simulink model "uav_control_ASMC"  (R2023a)
settings: Solver=FixedStepAuto  StartTime=0.0  StopTime=50  FixedStep=1e-3
undefined symbols (not defined in the file): C_SMC, control_form_LagrangeSimplified_forces, D_rot, D_transl, eulerlimit, g, J1, J2, J3, Jr, k1, k2, k3, k_phi, K_SMC, k_theta, m, Matrix_Force2angular_velocity, R
libraries: simulink x18, control_form_LagrangeSimplified x1
settings Model: Creator=Alex  LastModifiedBy=Alex

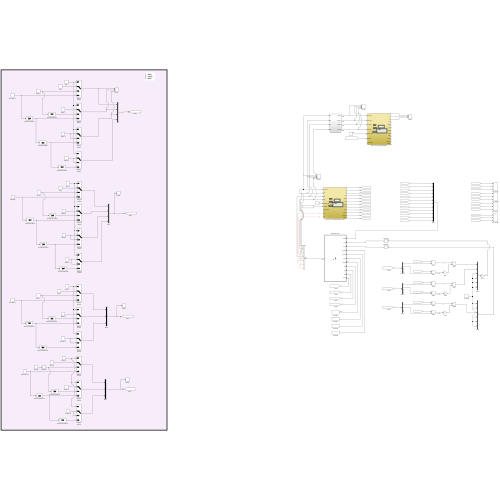
[thumbnail: Simulink's stored preview of the top-level diagram]
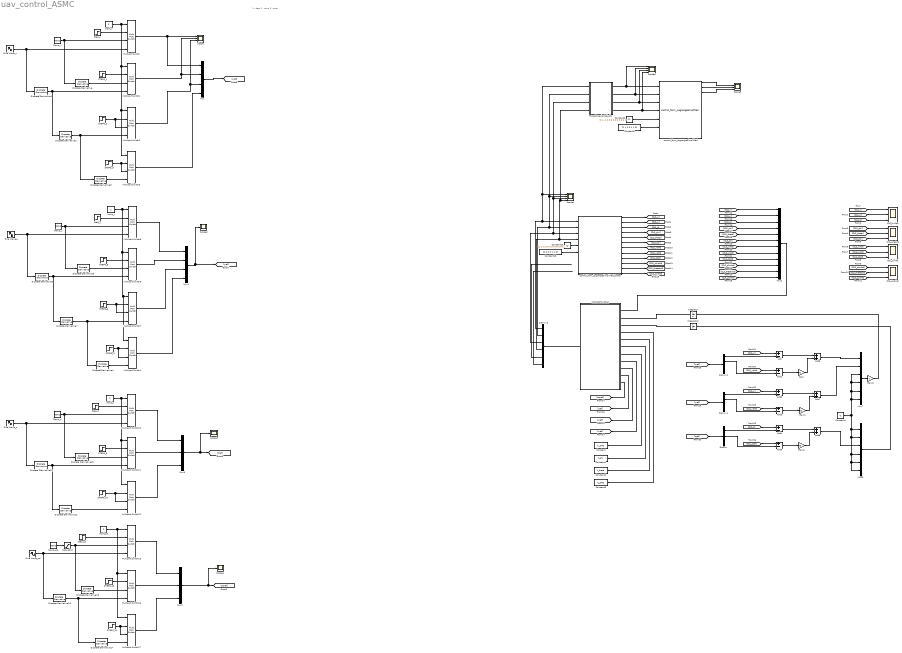
== system uav_control_ASMC ==
  note: 1 - step
      | 2 - ramp
      | 3 - else
  Add{,1..5} (6 alike) : Sum  Inputs=+-
  Add6 : Sum
  Add7 : Sum
  Add8 : Sum
  CNL_AngPos : Scope  NumInputPorts=3
  CNL_AngVel : Scope  NumInputPorts=3
  CNL_LinPos : Scope  NumInputPorts=3
  CNL_LinVel : Scope  NumInputPorts=3
  Constant : Constant  Value=K_SMC
  Constant1 : Constant  Value=k_phi
  Constant18 : Constant  Value=[1 0 0 0 1 1 0]
  Constant19 : Constant  Value=[1 1 -1 0 0 0 0 0 0 0 0 0 ]
  Constant2 : Constant  Value=k_theta
  Constant3 : Constant  Value=C_SMC
  Constant4 : Constant  Value=0
  Constant5 : Constant  Value=[1 1 0 0 1 1 0]
  Constant6 : Constant  Value=[1 1 -1 0 0 0 0 0 0 0 0 0 ]
  Demux : Demux  Outputs=3
  Demux1 : Demux
  Demux2 : Demux
  Demux3 : Demux  Outputs=6
  Discrete Derivative{,1..7,10..12,15..17} (14 alike) : simulink/Discrete/Discrete Derivative  gainval=1.0  ICPrevScaledInput=0.0  OutMin=[]  OutMax=[]  OutDataType=fixdt(1, 16)  OutScaling=2^-10  DoSatur=off
  Force2AngularVelocity : Subsystem
  Gain : Gain  Gain=k1
  Gain1 : Gain  Gain=k2
  Gain2 : Gain  Gain=k3
  Gain3 : Gain  Gain=-1
  Input_psi : Constant
  Input_x : Constant
  Input_y : Constant
  Input_z : Constant
  Integrator : Integrator
  Integrator1 : Integrator
  MATLAB Function : MATLAB Function  TreatAsAtomicUnit=on
  Multiport Switch{,1..7,10..12,15..17} (14 alike) : MultiPortSwitch  SaturateOnIntegerOverflow=off  InputSameDT=off
  Mux : Mux
  Mux1 : Mux
  Mux2 : Mux  Inputs=12
  Mux3 : Mux  Inputs=3
  Mux5 : Mux  Inputs=3
  Mux7 : Mux  Inputs=6
  Mux8 : Mux  Inputs=6
  Ramp_psi : simulink/Sources/Ramp  slope=0.2  start=0  InitialOutput=0
  Ramp_x : simulink/Sources/Ramp  slope=1  start=0  InitialOutput=1
  Ramp_y : simulink/Sources/Ramp  slope=1  start=0  InitialOutput=0
  Ramp_z : simulink/Sources/Ramp  slope=-5  start=0  InitialOutput=0
  STEP0_{1..6,9..10,13..14} (10 alike) : Step  Time=0  After=0  SampleTime=0
  Saturation : Saturate  UpperLimit=pi  LowerLimit=-pi
  Scope : Scope  NumInputPorts=3
  Scope1 : Scope  NumInputPorts=4
  Scope2 : Scope
  Scope3 : Scope
  Scope4 : Scope
  Scope5 : Scope  NumInputPorts=3
  Scope6 : Scope  NumInputPorts=4
  Sine Wave_psi : Sin  SampleTime=0
  Sine Wave_x : Sin  Frequency=0.5  SampleTime=0
  Sine Wave_y : Sin  Amplitude=3  Bias=5  SampleTime=0
  Sine Wave_z : Sin  Amplitude=3  Bias=-5  SampleTime=0
  Step_psi : Step  Time=0  SampleTime=0
  Step_x : Step  Time=0  After=5  SampleTime=0
  Step_y : Step  Time=0  After=5  SampleTime=0
  Step_z : Step  Time=0  After=-7  SampleTime=0
  control_form_LagrangeSimplified : control_form_LagrangeSimplified/control_form_LagrangeSimplified  SystemSampleTime=-1  VariantActivationTime=update diagram  Latency=0  AutoFrameSizeCalculation=off
  control_form_LagrangeSimplified_forces : Subsystem  AncestorBlock=control_form_LagrangeSimplified_forces/control_form_LagrangeSimplified_forces
  wires:
  Step_x/1 -> Multiport Switch/2
  Mux/1 -> [xref]
  Mux1/1 -> [yref], Scope2/1
  Step_psi/1 -> Multiport Switch15/2
  Mux3/1 -> Scope4/1, [psiref]
  Ramp_x/1 -> Discrete Derivative/1, Multiport Switch/3
  Sine Wave_x/1 -> Multiport Switch/4, Discrete Derivative1/1
  Input_x/1 -> Multiport Switch3/1, Multiport Switch2/1, Multiport Switch1/1, Multiport Switch/1
  STEP0_1/1 -> Multiport Switch1/2
  Discrete Derivative/1 -> Multiport Switch1/3
  Discrete Derivative1/1 -> Multiport Switch1/4, Discrete Derivative2/1
  STEP0_2/1 -> Multiport Switch2/3, Multiport Switch2/2
  Discrete Derivative2/1 -> Discrete Derivative3/1, Multiport Switch2/4
  Multiport Switch/1 -> Mux/1, Scope/1
  Multiport Switch1/1 -> Mux/2, Scope/2
  Multiport Switch2/1 -> Mux/3, Scope/3
  Multiport Switch7/1 -> Mux1/3
  Multiport Switch6/1 -> Mux1/2
  Multiport Switch5/1 -> Mux1/1
  Discrete Derivative7/1 -> Discrete Derivative4/1, Multiport Switch7/4
  STEP0_6/1 -> Multiport Switch7/2, Multiport Switch7/3
  Discrete Derivative6/1 -> Discrete Derivative7/1, Multiport Switch6/4
  Discrete Derivative5/1 -> Multiport Switch6/3
  STEP0_5/1 -> Multiport Switch6/2
  Input_y/1 -> Multiport Switch4/1, Multiport Switch7/1, Multiport Switch6/1, Multiport Switch5/1
  Sine Wave_y/1 -> Discrete Derivative6/1, Multiport Switch5/4
  Ramp_y/1 -> Multiport Switch5/3, Discrete Derivative5/1
  Step_y/1 -> Multiport Switch5/2
  Step_z/1 -> Multiport Switch10/2
  Ramp_z/1 -> Discrete Derivative10/1, Multiport Switch10/3
  Sine Wave_z/1 -> Multiport Switch10/4, Discrete Derivative11/1
  Input_z/1 -> Multiport Switch12/1, Multiport Switch11/1, Multiport Switch10/1
  STEP0_9/1 -> Multiport Switch11/2
  Discrete Derivative10/1 -> Multiport Switch11/3
  Discrete Derivative11/1 -> Multiport Switch11/4, Discrete Derivative12/1
  STEP0_10/1 -> Multiport Switch12/3, Multiport Switch12/2
  Discrete Derivative12/1 -> Multiport Switch12/4
  Multiport Switch10/1 -> Mux5/1
  Multiport Switch11/1 -> Mux5/2
  Multiport Switch12/1 -> Mux5/3
  Mux5/1 -> Scope3/1, [zref]
  Input_psi/1 -> Multiport Switch17/1, Multiport Switch16/1, Multiport Switch15/1
  Ramp_psi/1 -> Saturation/1
  Saturation/1 -> Discrete Derivative15/1, Multiport Switch15/3
  Sine Wave_psi/1 -> Discrete Derivative16/1, Multiport Switch15/4
  STEP0_13/1 -> Multiport Switch16/2
  Discrete Derivative15/1 -> Multiport Switch16/3
  Discrete Derivative16/1 -> Discrete Derivative17/1, Multiport Switch16/4
  STEP0_14/1 -> Multiport Switch17/3, Multiport Switch17/2
  Discrete Derivative17/1 -> Multiport Switch17/4
  Multiport Switch15/1 -> Mux3/1
  Multiport Switch16/1 -> Mux3/2
  Multiport Switch17/1 -> Mux3/3
  control_form_LagrangeSimplified_forces/1(x) -> [CLS_x]
  control_form_LagrangeSimplified_forces/2(y) -> [CLS_y]
  control_form_LagrangeSimplified_forces/3(z) -> [CLS_z]
  control_form_LagrangeSimplified_forces/4(phi) -> [CLS_phi]
  control_form_LagrangeSimplified_forces/5(theta) -> [CLS_theta]
  control_form_LagrangeSimplified_forces/6(psi) -> [CLS_psi]
  control_form_LagrangeSimplified_forces/7(xdot) -> [CLS_xdot]
  control_form_LagrangeSimplified_forces/8(ydot) -> [CLS_ydot]
  control_form_LagrangeSimplified_forces/9(zdot) -> [CLS_zdot]
  control_form_LagrangeSimplified_forces/10(phidot) -> [CLS_phidot]
  control_form_LagrangeSimplified_forces/11(thetadot) -> [CLS_thetadot]
  control_form_LagrangeSimplified_forces/12(psidot) -> [CLS_psidot]
  [CLS_x] -> Mux2/1
  [CLS_x] -> CNL_LinPos/1
  [CLS_y] -> Mux2/2
  [CLS_xdot] -> CNL_LinVel/1
  [CLS_psidot] -> Mux2/12
  [CLS_zdot] -> Mux2/9
  [CLS_thetadot] -> CNL_AngVel/2
  [CLS_phi] -> CNL_AngPos/1
  [CLS_ydot] -> CNL_LinVel/2
  [CLS_psidot] -> CNL_AngVel/3
  Mux2/1 -> MATLAB Function/1(states)
  [CLS_thetadot] -> Mux2/11
  [CLS_theta] -> CNL_AngPos/2
  [CLS_phidot] -> Mux2/10
  [CLS_theta] -> Mux2/5
  [CLS_z] -> Mux2/3
  [CLS_zdot] -> CNL_LinVel/3
  [CLS_ydot] -> Mux2/8
  [CLS_xdot] -> Mux2/7
  [CLS_psi] -> Mux2/6
  [CLS_phi] -> Mux2/4
  [CLS_y] -> CNL_LinPos/2
  [CLS_phidot] -> CNL_AngVel/1
  [CLS_psi] -> CNL_AngPos/3
  [CLS_z] -> CNL_LinPos/3
  Constant19/1 -> control_form_LagrangeSimplified_forces/5(initial_value)
  Constant18/1 -> control_form_LagrangeSimplified_forces/6(enables)
  Constant/1 -> MATLAB Function/7(K_SMC)
  Constant1/1 -> MATLAB Function/6(k_phi)
  Constant2/1 -> MATLAB Function/5(k_theta)
  Constant3/1 -> MATLAB Function/4(C_SMC)
  [psiref] -> MATLAB Function/11(psiref)
  [yref] -> MATLAB Function/9(yref)
  [zref] -> MATLAB Function/10(zref)
  [xref] -> MATLAB Function/8(xref)
  Integrator/1 -> MATLAB Function/2(v_hat)
  Integrator1/1 -> MATLAB Function/3(fr_hat)
  [zref] -> Demux/1
  [yref] -> Demux1/1
  [xref] -> Demux2/1
  [CLS_x] -> Add/1
  Demux2/1 -> Add/2
  [CLS_xdot] -> Add1/1
  Demux2/2 -> Add1/2
  Demux1/2 -> Add3/2
  [CLS_ydot] -> Add3/1
  Demux1/1 -> Add2/2
  [CLS_y] -> Add2/1
  [CLS_z] -> Add4/1
  Demux/1 -> Add4/2
  [CLS_zdot] -> Add5/1
  Demux/2 -> Add5/2
  Add/1 -> Add6/1  "ex"
  Add1/1 -> Gain/1  "ex_dot"
  Gain/1 -> Add6/2
  Add6/1 -> Mux7/1
  Add2/1 -> Add7/1  "ey"
  Add3/1 -> Gain1/1  "ey_dot"
  Gain1/1 -> Add7/2
  Add7/1 -> Mux7/2
  Add4/1 -> Add8/1  "ez"
  Add5/1 -> Gain2/1  "ez_dot"
  Gain2/1 -> Add8/2
  Add8/1 -> Mux8/3
  Constant4/1 -> Mux7/4, Mux7/3, Mux7/5, Mux7/6, Mux8/6, Mux8/5, Mux8/4, Mux8/2, Mux8/1
  Mux7/1 -> Gain3/1
  Mux8/1 -> Integrator1/1
  Gain3/1 -> Integrator/1
  Multiport Switch3/1 -> Mux/4
  Discrete Derivative3/1 -> Multiport Switch3/4
  STEP0_3/1 -> Multiport Switch3/3, Multiport Switch3/2
  Multiport Switch4/1 -> Mux1/4
  Discrete Derivative4/1 -> Multiport Switch4/4
  STEP0_4/1 -> Multiport Switch4/3, Multiport Switch4/2
  MATLAB Function/1(u) -> Demux3/1
  Demux3/1 -> Force2AngularVelocity/1(u1), Scope1/1, control_form_LagrangeSimplified_forces/1(F_thrust)
  Demux3/2 -> Force2AngularVelocity/2(u2), Scope1/2, control_form_LagrangeSimplified_forces/2(M1)
  Demux3/3 -> Force2AngularVelocity/3(u3), Scope1/3, control_form_LagrangeSimplified_forces/3(M2)
  Demux3/4 -> control_form_LagrangeSimplified_forces/4(M3), Force2AngularVelocity/4(u4), Scope1/4
  Demux3/5 -> ?
  Demux3/6 -> ?
  Force2AngularVelocity/1(omega_f) -> Scope6/1, control_form_LagrangeSimplified/1  "front"
  Force2AngularVelocity/2(omega_b) -> Scope6/2, control_form_LagrangeSimplified/2  "back"
  Force2AngularVelocity/3(omega_l) -> Scope6/3, control_form_LagrangeSimplified/3  "left"
  Force2AngularVelocity/4(omega_r) -> Scope6/4, control_form_LagrangeSimplified/4  "right"
  control_form_LagrangeSimplified/1 -> Scope5/1
  control_form_LagrangeSimplified/2 -> Scope5/2
  control_form_LagrangeSimplified/3 -> Scope5/3
  Constant5/1 -> control_form_LagrangeSimplified/6
  Constant6/1 -> control_form_LagrangeSimplified/5

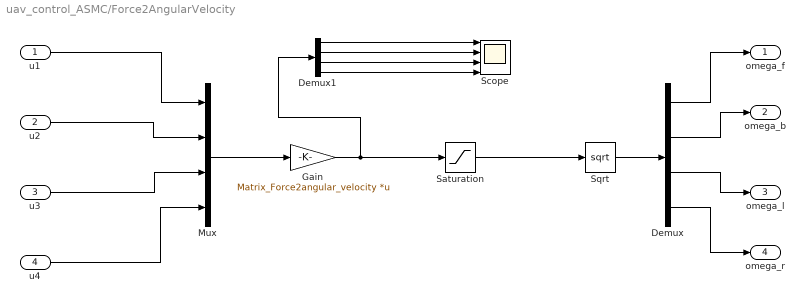
== system uav_control_ASMC/Force2AngularVelocity ==
  u1 : Inport
  u2 : Inport  Port=2
  u3 : Inport  Port=3
  u4 : Inport  Port=4
  Demux : Demux
  Demux1 : Demux
  Gain : Gain  Gain=Matrix_Force2angular_velocity  Multiplication=Matrix(K*u)
  Mux : Mux
  Saturation : Saturate  UpperLimit=inf  LowerLimit=0
  Scope : Scope  NumInputPorts=4
  Sqrt : Sqrt
  omega_f : Outport
  omega_b : Outport  Port=2
  omega_l : Outport  Port=3
  omega_r : Outport  Port=4
  wires:
  u3/1 -> Mux/3
  u2/1 -> Mux/2
  u4/1 -> Mux/4
  u1/1 -> Mux/1
  Mux/1 -> Gain/1
  Sqrt/1 -> Demux/1
  Demux/3 -> omega_l/1
  Demux/2 -> omega_b/1
  Demux/4 -> omega_r/1
  Demux/1 -> omega_f/1
  Demux1/1 -> Scope/1
  Demux1/2 -> Scope/2
  Demux1/3 -> Scope/3
  Demux1/4 -> Scope/4
  Gain/1 -> Saturation/1, Demux1/1
  Saturation/1 -> Sqrt/1

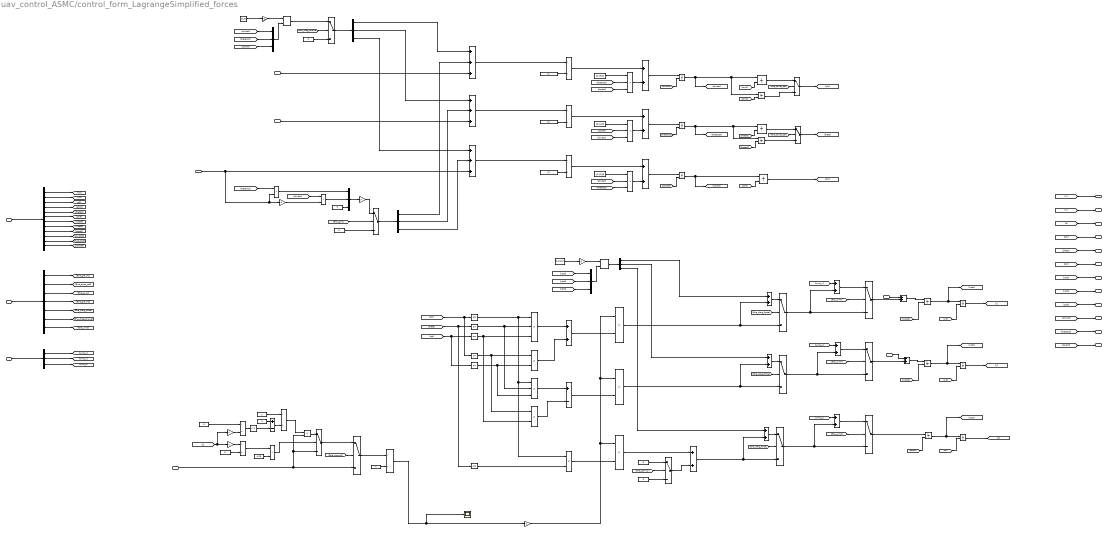
== system uav_control_ASMC/control_form_LagrangeSimplified_forces ==
  note: Drag force
  note: Translational dynamics
  note: Simplified Euler equations of motion
      | Rotational dynamics
  note: Gyro
  note: Drag torque
  note: Ground
  F_thrust : Inport
  M1 : Inport  Port=2
  M2 : Inport  Port=3
  M3 : Inport  Port=4
  initial_value : Inport  Port=5
  enables : Inport  Port=6
  wind_power : Inport  Port=7
  u5 : Inport  Port=8
  u6 : Inport  Port=9
  Add{,1,3..5,18,20..24,33..34} (13 alike) : Sum
  Add10 : Sum  Inputs=+++
  Add11 : Sum  Inputs=+++
  Add19 : Sum  Inputs=+-
  Add25 : Sum  Inputs=+++
  Add26 : Sum  Inputs=+-
  Constant : Constant  Value=J1
  Constant1 : Constant  Value=J2
  Constant10 : Constant  Value=R
  Constant{9,11,13,20} (4 alike) : Constant  Value=0
  Constant12 : Constant  Value=D_rot
  Constant14 : Constant  Value=0.25
  Constant15 : Constant  Value=R
  Constant16 : Constant
  Constant17 : Constant
  Constant19 : Constant  Value=D_transl
  Constant2 : Constant  Value=J3
  Constant21 : Constant  Value=g
  Constant3 : Constant  Value=(J2-J3)/J1
  Constant4 : Constant  Value=(J3-J1)/J2
  Constant5 : Constant  Value=(J1-J2)/J3
  Constant6 : Constant  Value=m
  Cos : Trigonometry  Operator=cos
  Cos1 : Trigonometry  Operator=cos
  Demux : Demux  Outputs=12
  Demux1 : Demux  Outputs=7
  Demux{2..3,5..6} (4 alike) : Demux  Outputs=3
  Divide{,1..2,5..8} (7 alike) : Product  Inputs=*/
  Gain10 : Gain  Gain=4
  Gain{6,8..9,12..13} (5 alike) : Gain  Gain=-1
  Gain7 : Gain  Gain=Jr
  Integrator{,1..3,7..11,13..14} (11 alike) : Integrator  InitialConditionSource=external
  Integrator4 : Integrator  InitialConditionSource=external  LimitOutput=on  UpperSaturationLimit=eulerlimit  LowerSaturationLimit=-eulerlimit
  Integrator5 : Integrator  InitialConditionSource=external  LimitOutput=on  UpperSaturationLimit=eulerlimit  LowerSaturationLimit=-eulerlimit
  Integrator6 : Integrator  InitialConditionSource=external  LimitOutput=on  UpperSaturationLimit=pi  LowerSaturationLimit=-pi
  Mux : Mux  Inputs=3
  Mux1 : Mux  Inputs=3
  Mux3 : Mux  Inputs=3
  Product16 : Product  Multiplication=Matrix(*)
  Product{17..19,28,30..34} (9 alike) : Product
  Product{4..6,27,29} (5 alike) : Product  Inputs=3
  Product35 : Product  Multiplication=Matrix(*)
  Relational Operator : RelationalOperator  Operator=>  OutDataTypeStr=boolean  RndMeth=Simplest  InputSameDT=off
  Scope1 : Scope
  Sin12 : Trigonometry
  Sin13 : Trigonometry  Operator=cos
  Sin14 : Trigonometry
  Sin15 : Trigonometry
  Square : Math  Operator=square
  Switch{,1..5,11..17} (13 alike) : Switch  Criteria=u2 ~= 0  SaturateOnIntegerOverflow=off  InputSameDT=off
  x : Outport
  y : Outport  Port=2
  z : Outport  Port=3
  phi : Outport  Port=4
  theta : Outport  Port=5
  psi : Outport  Port=6
  xdot : Outport  Port=7
  ydot : Outport  Port=8
  zdot : Outport  Port=9
  phidot : Outport  Port=10
  thetadot : Outport  Port=11
  psidot : Outport  Port=12
  wires:
  [Ena_drag_force] -> Switch13/2
  Add20/1 -> Add21/2, Switch13/3
  Add21/1 -> Switch13/1
  Mux3/1 -> Product35/2
  [zdot] -> Mux3/3
  [xdot] -> Mux3/1
  Gain13/1 -> Product35/1
  Constant19/1 -> Gain13/1
  [ydot] -> Mux3/2
  Add22/1 -> Switch14/1
  Product33/1 -> Switch14/3, Add22/2
  [Ena_drag_force] -> Switch14/2
  [Ena_drag_force] -> Switch15/2
  Product32/1 -> Switch15/3, Add23/2
  Add23/1 -> Switch15/1
  Product35/1 -> Demux6/1
  Demux6/2 -> Add22/1
  Demux6/3 -> Add21/1
  Switch13/1 -> Add34/2, Switch16/3
  Switch14/1 -> Add33/2, Switch17/3
  Switch15/1 -> Add24/2, Switch12/3
  [Ena_wind] -> Switch17/2
  [Ena_wind] -> Switch16/2
  [Ena_wind] -> Switch12/2
  Add24/1 -> Switch12/1
  Add33/1 -> Switch17/1
  Add34/1 -> Switch16/1
  [wind_x] -> Add24/1
  [wind_y] -> Add33/1
  [wind_z] -> Add34/1
  Demux6/1 -> Add23/1
  Switch11/1 -> Add20/2  "gravity"
  [Ena_gravity] -> Switch11/2
  Constant21/1 -> Switch11/1
  Constant20/1 -> Switch11/3
  Gain12/1 -> Product34/1, Product33/1, Product32/1
  Cos1/1 -> Product30/2, Product27/3
  Product27/1 -> Add18/1
  [x0] -> Integrator14/2
  Integrator13/1 -> [y]
  [theta] -> Sin13/1, Sin14/1
  Add18/1 -> Product32/2
  [psi] -> Cos1/1, Sin12/1
  Product31/1 -> Product34/2
  Integrator11/1 -> [z]
  Integrator10/1 -> Integrator11/1, [zdot]
  Product34/1 -> Add20/1
  [zdot0] -> Integrator10/2
  [xdot0] -> Integrator3/2
  Product28/1 -> Add18/2
  Add19/1 -> Product33/2
  Integrator3/1 -> Integrator14/1, [xdot]
  Sin13/1 -> Product31/2
  [y0] -> Integrator13/2
  Integrator14/1 -> [x]
  [ydot0] -> Integrator9/2
  Product29/1 -> Add19/1
  Cos/1 -> Product31/1, Product29/1, Product27/1
  Sin14/1 -> Product29/2, Product27/2
  [phi] -> Sin15/1, Cos/1
  Switch16/1 -> Integrator10/1
  Switch17/1 -> Add1/2
  Integrator9/1 -> Integrator13/1, [ydot]
  Sin12/1 -> Product29/3, Product28/2
  Sin15/1 -> Product30/1, Product28/1
  [z0] -> Integrator11/2
  Product30/1 -> Add19/2
  Switch12/1 -> Add/2
  Demux5/3 -> [wind_z]
  Demux5/2 -> [wind_y]
  Demux5/1 -> [wind_x]
  Demux2/3 -> Add10/1
  Demux2/1 -> Add25/1
  Constant17/1 -> Divide8/1
  Add26/1 -> Divide8/2
  Divide8/1 -> Product19/1
  Constant16/1 -> Add26/1
  Square/1 -> Add26/2
  Divide7/1 -> Square/1
  Gain10/1 -> Divide7/2
  Constant15/1 -> Divide7/1
  Product19/1 -> Switch4/1
  Constant14/1 -> Relational Operator/2
  Relational Operator/1 -> Switch4/2
  Constant10/1 -> Divide6/2
  Divide6/1 -> Relational Operator/1
  Gain9/1 -> Divide6/1
  [z] -> Gain9/1, Gain10/1
  Switch4/1 -> Switch2/1
  Switch2/1 -> Divide5/1  "ground"
  [Ena_ground] -> Switch2/2
  Demux2/2 -> Add11/1
  Demux3/1 -> Add25/2
  Demux3/2 -> Add11/2
  Demux3/3 -> Add10/2
  Gain8/1 -> Product18/2
  Gain7/1 -> Switch1/1
  Mux1/1 -> Gain7/1
  Constant13/1 -> Mux1/3
  Product18/1 -> Mux1/2
  Product17/1 -> Mux1/1
  [phidot] -> Product18/1
  [thetadot] -> Product17/1
  Switch1/1 -> Demux3/1  "gyro"
  Switch3/1 -> Demux2/1  "drag_torque"
  Product16/1 -> Switch3/1
  Mux/1 -> Product16/2
  [psidot] -> Mux/3
  [phidot] -> Mux/1
  [thetadot] -> Mux/2
  Gain6/1 -> Product16/1
  Constant12/1 -> Gain6/1
  Constant11/1 -> Switch1/3
  Constant9/1 -> Switch3/3
  [Ena_drag_torque] -> Switch3/2
  [Ena_gyro] -> Switch1/2
  Add25/1 -> Divide/1  "tau1"
  Add11/1 -> Divide1/1  "tau2"
  Add10/1 -> Divide2/1  "tau3"
  wind_power/1 -> Demux5/1
  Demux1/7 -> [Ena_wind]
  Demux1/6 -> [Ena_drag_torque]
  Demux1/5 -> [Ena_drag_force]
  Demux1/4 -> [Ena_ground]
  Demux1/3 -> [Ena_gyro]
  Demux1/1 -> [Ena_gravity]
  enables/1 -> Demux1/1
  [psidot0] -> Integrator2/2
  [thetadot0] -> Integrator1/2
  [phidot0] -> Integrator/2
  Demux/12 -> [psidot0]
  Demux/11 -> [thetadot0]
  Demux/10 -> [phidot0]
  Demux/9 -> [zdot0]
  Demux/8 -> [ydot0]
  Demux/7 -> [xdot0]
  Demux/6 -> [psi0]
  Demux/5 -> [theta0]
  Demux/4 -> [phi0]
  Demux/3 -> [z0]
  Demux/2 -> [y0]
  Demux/1 -> [x0]
  initial_value/1 -> Demux/1
  Divide5/1 -> Gain12/1, Scope1/1
  [z] -> z/1
  [phi] -> phi/1
  [theta] -> theta/1
  [psi] -> psi/1
  [xdot] -> xdot/1
  [ydot] -> ydot/1
  [zdot] -> zdot/1
  [phidot] -> phidot/1
  [thetadot] -> thetadot/1
  [psidot] -> psidot/1
  [y] -> y/1
  [x] -> x/1
  Constant6/1 -> Divide5/2
  F_thrust/1 -> Switch2/3, Switch4/3, Product19/2  "Fa"
  [thetadot] -> Product6/3
  [phidot] -> Product6/2
  [phidot] -> Product5/3
  [psidot] -> Product5/2
  [psidot] -> Product4/3
  [thetadot] -> Product4/2
  Add5/1 -> Integrator2/1
  Add4/1 -> Integrator1/1
  Add3/1 -> Integrator/1
  Constant5/1 -> Product6/1
  Constant4/1 -> Product5/1
  Constant3/1 -> Product4/1
  Product6/1 -> Add5/2
  Product5/1 -> Add4/2
  Product4/1 -> Add3/2
  Divide2/1 -> Add5/1
  Divide1/1 -> Add4/1
  Divide/1 -> Add3/1
  Constant2/1 -> Divide2/2
  Constant1/1 -> Divide1/2
  Constant/1 -> Divide/2
  M3/1 -> Product17/2, Gain8/1, Add10/3  "M3"
  M2/1 -> Add11/3  "M2"
  M1/1 -> Add25/3  "M1"
  Add/1 -> Integrator3/1
  u5/1 -> Add/1  "u5"
  Add1/1 -> Integrator9/1
  u6/1 -> Add1/1  "u6"
  Demux1/2 -> [Ena_euler_sat]
  Integrator8/1 -> Switch5/3  "phi_nolim"
  Integrator2/1 -> Integrator6/1, [psidot]  "psidot"
  Integrator1/1 -> [thetadot], Integrator5/1, Integrator7/1  "thetadot"
  Integrator/1 -> Integrator8/1, Integrator4/1, [phidot]  "phidot"
  [Ena_euler_sat] -> Switch/2
  [theta0] -> Integrator5/2
  Switch5/1 -> [phi]  "phi"
  Integrator4/1 -> Switch5/1  "phi_lim"
  [theta0] -> Integrator7/2
  Integrator7/1 -> Switch/3  "theta_nolim"
  Integrator5/1 -> Switch/1  "theta_lim"
  [psi0] -> Integrator6/2
  [phi0] -> Integrator8/2
  Switch/1 -> [theta]  "theta"
  Integrator6/1 -> [psi]  "psi"
  [Ena_euler_sat] -> Switch5/2
  [phi0] -> Integrator4/2

== matlab function uav_control_ASMC/MATLAB Function ==
  data: states input; v_hat input; fr_hat input; C_SMC input; k_theta input; k_phi input; K_SMC input; xref input; yref input; zref input; psiref input; u output
function u = fcn_smc(states, v_hat, fr_hat, C_SMC, k_theta, k_phi, K_SMC, xref, yref, zref, psiref)
    arguments
        states (12,1) {mustBeNumeric}
        v_hat
        fr_hat
        C_SMC 
        k_theta
        k_phi
        K_SMC
        xref (4,1)
        yref (4,1)
        zref (3,1)
        psiref (3,1)

    end

 m=1.888;
 g=9.81;
 J1=1.453e-2;
 J2=1.453e-2;
 J3=2.884e-2;

 x=states(1);
 y=states(2);
 z=states(3);
 phi=states(4);
 theta=states(5);
 psi=states(6);
 xdot=states(7);
 ydot=states(8);
 zdot=states(9);
 phidot=states(10);
 thetadot=states(11);
 psidot=states(12);

 xdesired=xref(1);
 xdesired_dot=xref(2);
 ydesired=yref(1);
 ydesired_dot=yref(2);
 zdesired=zref(1);
 zdesired_dot=zref(2);
 psidesired=psiref(1);
 psidesired_dot=psiref(2);
 xdesired_d_dot=xref(3);
 ydesired_d_dot=yref(3);
 zdesired_d_dot=zref(3);
 psidesired_d_dot=psiref(3);


 ex=x-xdesired;
 ex_dot=xdot-xdesired_dot;
 ey=y-ydesired;
 ey_dot=ydot-ydesired_dot;
 ez=z-zdesired;
 ez_dot=zdot-zdesired_dot;
 epsi=psi-psidesired;
 epsi_dot=psidot-psidesired_dot;
 
 % x_d_dot=-1/m*(cos(phi)*sin(theta)*cos(psi)+sin(phi)*sin(psi))*u1; 
 % y_d_dot=-1/m*(cos(phi)*sin(theta)*sin(psi)-sin(phi)*cos(psi))*u1;
 % 
 % x_dots_3=-1/m*(-phidot*sin(phi)*sin(theta)*cos(psi)+thetadot*cos(phi)*cos(theta)*cos(psi)-...
 %     psidot*cos(phi)*sin(theta)*sin(psi)+phidot*cos(phi)*sin(psi)+psidot*sin(phi)*cos(psi))*u1+u1dot*-1/m*(cos(phi)*sin(theta)*cos(psi)+sin(phi)*sin(psi));
 % y_dots_3=-1/m*(-phidot*sin(phi)*sin(theta)*sin(psi)+thetadot*cos(phi)*cos(theta)*sin(psi)+...
 %     psidot*cos(phi)*sin(theta)*cos(psi)-phidot*cos(phi)*cos(psi)+psidot*sin(phi)*sin(psi))*u1+u1dot*-1/m*(cos(phi)*sin(theta)*sin(psi)-sin(phi)*cos(psi));

 x_d_dot=-1/m*(cos(phi)*sin(theta)*cos(psi)+sin(phi)*sin(psi)); 
 y_d_dot=-1/m*(cos(phi)*sin(theta)*sin(psi)-sin(phi)*cos(psi));

 x_dots_3=-1/m*(-phidot*sin(phi)*sin(theta)*cos(psi)+thetadot*cos(phi)*cos(theta)*cos(psi)-...
     psidot*cos(phi)*sin(theta)*sin(psi)+phidot*cos(phi)*sin(psi)+psidot*sin(phi)*cos(psi));
 y_dots_3=-1/m*(-phidot*sin(phi)*sin(theta)*sin(psi)+thetadot*cos(phi)*cos(theta)*sin(psi)+...
     psidot*cos(phi)*sin(theta)*cos(psi)-phidot*cos(phi)*cos(psi)+psidot*sin(phi)*sin(psi));

 thetadesired=ex_dot+k_theta*ex;
 thetadesired_dot=(x_d_dot-xref(3))+k_theta*ex_dot;
 phidesired=ey_dot+k_phi*ey;
 phidesired_dot=(y_d_dot-yref(3))+k_phi*ey_dot;

 thetadesired_d_dot=(x_dots_3-xref(4))+k_theta*(x_d_dot-xdesired_d_dot);
 phidesired_d_dot=(y_dots_3-yref(4))+k_phi*(y_d_dot-ydesired_d_dot);
 %

 
 ephi=phi-phidesired;
 ephi_dot=phidot-phidesired_dot;
 etheta=theta-thetadesired;
 etheta_dot=thetadot-thetadesired_dot;

 e=[ex ey ez ephi etheta epsi]';
 e_dot=[ex_dot ey_dot ez_dot ephi_dot etheta_dot epsi_dot]';
 
 s=e_dot+K_SMC*e;

 G=[x_d_dot,0,0,0,1,0;...
     y_d_dot,0,0,0,0,1;
     -1/m*cos(phi)*cos(theta),0,0,0,0,0;
     0,1/J1,0,0,0,0;
     0,0,1/J2,0,0,0;
     0,0,0,1/J3,0,0];
 Ginv=inv(G);

 f=[0;0;g;(J2-J3)/J1*thetadot*psidot;(J3-J1)/J2*psidot*phidot;(J1-J2)/J3*phidot*thetadot];
 state_desired_d_dot=[xdesired_d_dot ydesired_d_dot zdesired_d_dot phidesired_d_dot thetadesired_d_dot psidesired_d_dot]';
u=Ginv*(-f+v_hat-fr_hat+state_desired_d_dot-K_SMC*e_dot-diag([C_SMC(1),C_SMC(2),C_SMC(3),C_SMC(4),C_SMC(5),C_SMC(6)])*[sign(s(1)) sign(s(2)) sign(s(3)) sign(s(4)) sign(s(5)) sign(s(6))]');
% u=Ginv*(-f-fr_hat+state_desired_d_dot-K_SMC*e_dot-diag([C_SMC(1),C_SMC(2),C_SMC(3),C_SMC(4),C_SMC(5),C_SMC(6)])*[saturation_f(s(1)/0.3) saturation_f(s(2)/0.3) saturation_f(s(3)/0.3) saturation_f(s(4)/0.3) saturation_f(s(5)/0.3) saturation_f(s(6)/0.3)]');

 function out=saturation_f(x) 
    if(abs(x)<=1)
        out=x;
    else
        out=x/abs(x);
    end
 end
end
